simulink model "TrainingModel"  (R2024b)
settings: Solver=VariableStepAuto  StartTime=0.0  StopTime=1  RelTol=1e-3
libraries: dspobslib x1
settings Model: Creator=pvenupra  LastModifiedBy=alial

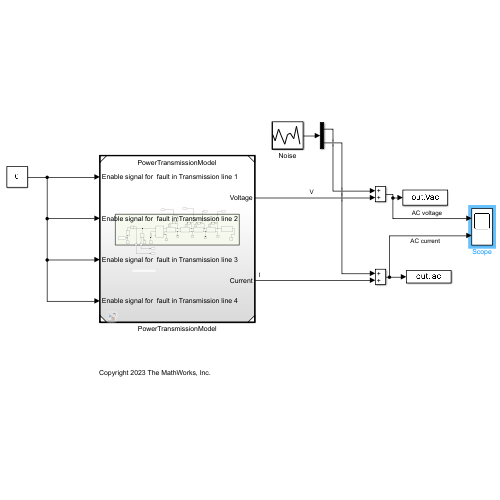
[thumbnail: Simulink's stored preview of the top-level diagram]
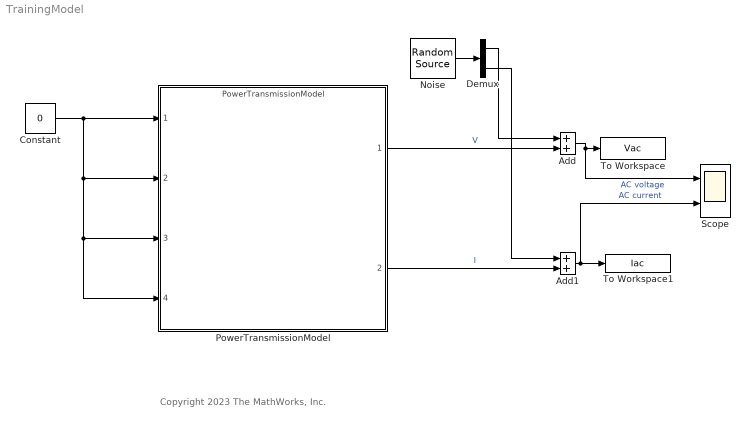
== system TrainingModel ==
  note: Copyright 2023 The MathWorks, Inc.
  Add : Sum
  Add1 : Sum
  Constant : Constant  Value=0  SampleTime=0.025
  Demux : Demux  Outputs=2
  Noise : dspobslib/Random Source  SrcType=Gaussian  NormMethod=Ziggurat  CltLength=12  MinVal=0  MaxVal=1  MeanVal=0  VarVal=[1000 .01]  RepMode=Specify seed  rawSeed=1  IsInherit=off  SampMode=Discrete  SampTime=1e-4  SampFrame=1  DataType=Double  OutComplex=Real  OutputFrames=on
  PowerTransmissionModel : ModelReference  ModelNameDialog=PowerTransmissionModel.slx  SimulationMode=Normal  ModelReferenceVersion=4.11
  Scope : Scope  NumInputPorts=2
  To Workspace : ToWorkspace  VariableName=Vac  SampleTime=-1
      settings: Save2DSignal=2-D array (concatenate along first dimension)
  To Workspace1 : ToWorkspace  VariableName=Iac  SampleTime=-1
      settings: Save2DSignal=2-D array (concatenate along first dimension)
  wires:
  Demux/2 -> Add1/1
  PowerTransmissionModel/2 -> Add1/2  "I"
  PowerTransmissionModel/1 -> Add/2  "V"
  Noise/1 -> Demux/1
  Add1/1 -> Scope/2, To Workspace1/1  "AC current"
  Demux/1 -> Add/1
  Add/1 -> Scope/1, To Workspace/1  "AC voltage"
  Constant/1 -> PowerTransmissionModel/4, PowerTransmissionModel/3, PowerTransmissionModel/2, PowerTransmissionModel/1
